simulink model "ThevinenIdentification_uding_ESCAndEst"  (R2021b)
settings: Solver=VariableStepAuto  StartTime=0.0  StopTime=300  FixedStep=0.01  MaxStep=1  RelTol=1e-4
undefined symbols (not defined in the file): sgn
libraries: simulink_extras x7, spsSeriesRLCBranchLib x4, spsBreakerLib x2, spsFourierLib x2, spsACVoltageSourceLib x1, simulink x1, spsGroundLib x1, spsControlledCurrentSourceLib x1, spsCurrentMeasurementLib x1, spsPowerLib x1, spsVoltageMeasurementLib x1, spspowerguiLib x1
settings Model: Creator=tahas  LastModifiedBy=tahas

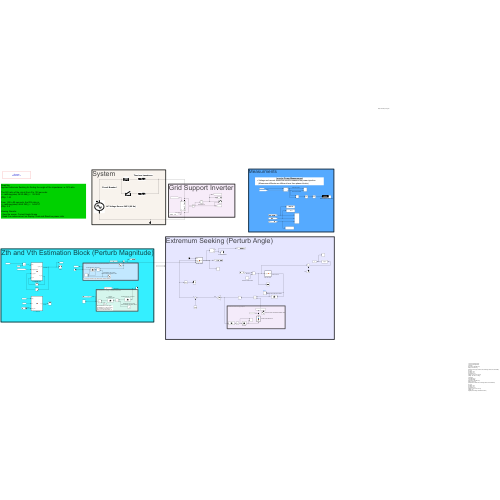
[thumbnail: Simulink's stored preview of the top-level diagram]
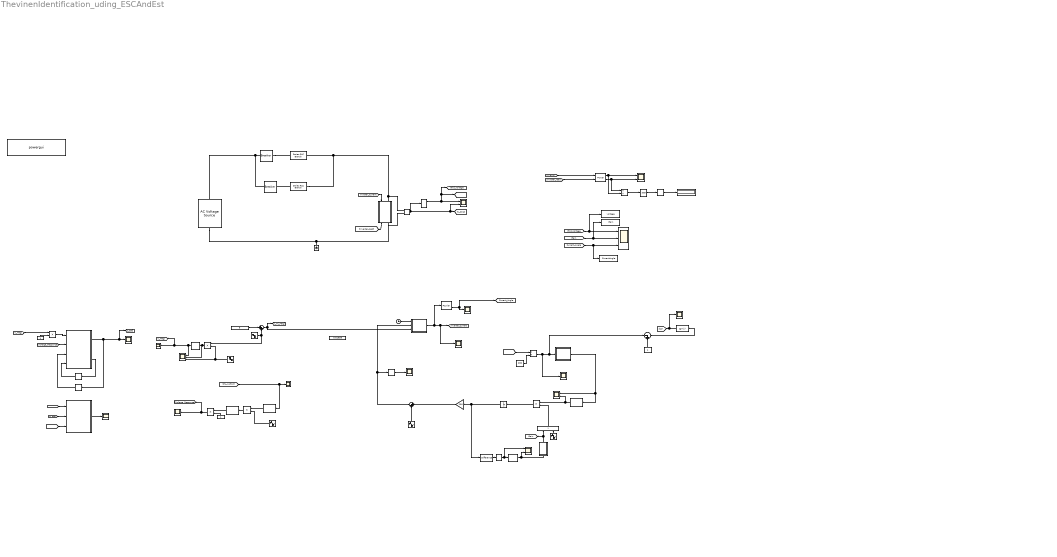
== system ThevinenIdentification_uding_ESCAndEst ==
  note: Zth and Vth Estimation Block (Perturb Magnitude)
  note: Grid Support Inverter (Current Source)
  note: After demodulation, the DC signal gets divided by 2, so we can multiply by 2 if needed (not needed here since input is also got divided by 2)
  note: Conditional Gain Change (Optional)
  note: System
  note: Measurments
  note: Extremum Seeking (Perturb Angle)
  note: Read Me:
      | Applies Extremum Seeking for finding the angle of the impedance i.e. R/X ratio.
      |
      | The R/X ratio of the circuit from 0 to 100 seconds:
      | >> rad2deg(atan(.343/0.484)) = 35.3243
      | |Zth|= 1.42
      |
      | From 105 to 90 seconds, the R/X ratio is:
      | >> rad2deg(atan(0.484/.343)) = 54.6757
      | |Zth|= 2.8
      |
      | Viewing Results:
      | - View the scope: Current Angle Scope
      | - Read the measurement on display: Real and Reactive power ratio
      |
      | Note:
      | Change filter to s/(s+1) and gain to 150 to visualize beautiful convergence
      | Change filter to s/(s+5) and gain to 200 to get quick convergence
  note: x=out.CurrentAngle.Time;
      | y=out.CurrentAngle.Data;
      | yyaxis left
      | h(1)=plot(x,y,'linewidth',2.0);
      | axis([13 34 -200 200])
      | ylabel('Current Angle','FontSize',32,'FontWeight','bold','Color','#0072BD')
      | ax = gca;
      | ax.XGrid = 'off';
      | ax.YGrid = 'on';
      | ax.FontSize = 32;
      | xticks([15 18 21 24 27 30 32])
      | yticks([ -180 -60 -30 0 180])
      | yyaxis right
      | x=out.Gain.Time;
      | y=out.Gain.Data;
      | h(2)=plot(x,y,'linewidth',2.0);
      | axis([13 34 -5 45])
      | ylabel('Gain','FontSize',32,'FontWeight','bold','Color','#D95319')
      | ax = gca;
      | ax.XGrid = 'off';
      | ax.YGrid = 'on';
      | ax.FontSize = 32;
      | xticks([15 18 21 24 27 30 33])
      | yticks([ 1 8])
      | legend('Current Angle','Demodulator Gain')
  note: Inverter Power Measurement
      | Voltage and current should be used to measure the power injection (Measuremnt Blocks are different here then phasor blocks)
  note: Circuit Breakerl
  note: Thevinen Impedance
  note: AC Voltage Source 245 V (60 Hz)
  note: For viewing the waveforms (the effect of filter and demodulation)
  note: Saving the 0.5 of ampliftude of applied perturbation
  note: The response on voltage of applied perturbation
  note: atan(.343/0.484) in degree
  " Intention: To separate DC part" : simulink_extras/Additional Linear/Transfer Fcn (with initial outputs)  N=[0 1]  D="[1  1]"  Y0=0  U0=0
  AC Voltage Source1 : spsACVoltageSourceLib/AC Voltage Source  Amplitude=245  Phase=0  Frequency=60  SampleTime=0  Measurements=None  BusType=swing  Pref=10e3  Qref=0  Qmin=-inf  Qmax=+inf
  Add1 : Sum  Inputs=|-+
  Atan1 : Trigonometry  Operator=atan
  Breaker1 : spsBreakerLib/Breaker  InitialState=1  SwitchingTimes=[105 195]  External=off  BreakerResistance=0.00000001  SnubberResistance=1e6  SnubberCapacitance=inf  Measurements=None  MoreParameters=on  NoBreakLoop=off
      settings: SourceProductBaseCode=PS
  Breaker3 : spsBreakerLib/Breaker  InitialState=0  SwitchingTimes=[100 200]  External=off  BreakerResistance=0.00000001  SnubberResistance=1e6  SnubberCapacitance=inf  Measurements=None  MoreParameters=on  NoBreakLoop=off
      settings: SourceProductBaseCode=PS
  Clock : Clock
  Complex to Magnitude-Angle : ComplexToMagnitudeAngle  Output=Magnitude
  "Conditional Gain Adjustment " : MATLAB Function  TreatAsAtomicUnit=on
  Current Angle Scope : Scope
  "Demodulation with the same signal as applied parturbation, Mag=1" : Sin  Frequency=10  SampleTime=0
  "Demodulation with the same signal as applied parturbation, Mag=1 " : Sin  Frequency=10  SampleTime=0
  Difference : simulink/Discrete/Difference  ICPrevInput=0  OutMin=[]  OutMax=[]  OutDataType=fixdt(1, 16)  OutScaling=2^-10  DoSatur=off
  Divide1 : Product  Inputs=*/
  Divide4 : Product  Inputs=*/
  Fcn2 : Fcn  Expr=sgn(u)
  Fourier at 60 Hz : spsFourierLib/Fourier  Freq=60  n=1  InInit=[0, 0]  Ts=0
      settings: SourceProductBaseCode=PS
  Fourier7 : spsFourierLib/Fourier  Freq=60  n=1  InInit=[0, 0]  Ts=0
      settings: SourceProductBaseCode=PS
  Gain : Gain  Gain=200
  Ground2 : spsGroundLib/Ground  LConnTagsString=a
  High pass filter (with initial outputs)1 : simulink_extras/Additional Linear/Transfer Fcn (with initial outputs)  N=[1 0]  D="[1  5]"  Y0=0  U0=0
  High pass filter with 1 rad cut off : simulink_extras/Additional Linear/Transfer Fcn (with initial outputs)  N=[1 0]  D="[1  1]"  Y0=0  U0=0
  Integrator1 : Integrator
  Inverter : Subsystem
  Low Pass : simulink_extras/Additional Linear/Transfer Fcn (with initial outputs)  N=[0 1]  D="[1  6]"  Y0=0  U0=0
  Low pass filter with 1 rad cut off : simulink_extras/Additional Linear/Transfer Fcn (with initial outputs)  N=[0 1]  D="[1  1]"  Y0=0  U0=0
  Normilizing voltage (peak) : Constant  Value=280
  P_Prev : Memory  InitialCondition=0.1
  Power : spsPowerLib/Power  Freq=60  Vinit=[1, 0]  Iinit=[1, 0]  Ts=0
      settings: SourceProductBaseCode=PS
  Product{1..3,5..7} (6 alike) : Product
  Radians to Degrees : simulink_extras/Transformations/Radians to Degrees
  Radians to Degrees2 : simulink_extras/Transformations/Radians to Degrees
  Real Power (watts)1 : Constant  Value=5
  Real Power (watts)2 : Constant
  Real Power (watts)3 : Constant
  Real Power (watts)4 : Constant  Value=0.61655
  "Real and Reactive power ratio " : Display
  Scope{1,5,12,14} (4 alike) : Scope  NumInputPorts=2
  Scope10 : Scope  NumInputPorts=3
  Scope{2..4,6..7,9,11} (7 alike) : Scope
  Scope15 : Scope  NumInputPorts=3
  Series RLC Branch1 : spsSeriesRLCBranchLib/Series RLC Branch  LConnTagsString=__new0  RConnTagsString=__new0  BranchType=RL  Resistance=12*0.343*40/100  Inductance=12*0.484/(2*pi*60) *40/100  SetiL0=off  InitialCurrent=0  Capacitance=1e-6  Setx0=off  InitialVoltage=0  Measurements=None
  Series RLC Branch7 : spsSeriesRLCBranchLib/Series RLC Branch  LConnTagsString=__new0  RConnTagsString=__new0  BranchType=RL  Resistance=6*0.484*40/100  Inductance=6*0.343/(2*pi*60)*40/100  SetiL0=off  InitialCurrent=0  Capacitance=1e-6  Setx0=off  InitialVoltage=0  Measurements=None
  Sine Wave (same as applied perturbation freq) : Sin  Frequency=5  SampleTime=0
  Sine Wave2 : Sin  Amplitude=0.01  Frequency=5  SampleTime=0
  Sine Wave5 : Sin  Amplitude=0.005  Frequency=10  SampleTime=0
  Sum1 : Sum  Inputs=|++
  Sum3 : Sum  Inputs=|++
  To Workspace : ToWorkspace  VariableName=voltage  SaveFormat=Timeseries  SampleTime=-1
  To Workspace1 : ToWorkspace  VariableName=Gain  SaveFormat=Timeseries  SampleTime=-1
  To Workspace2 : ToWorkspace  VariableName=CurrentAngle  SaveFormat=Timeseries  SampleTime=-1
  V1 : Scope
  V_th_Est Block : MATLAB Function  TreatAsAtomicUnit=on
  Volt_Var_Curve1 : MATLAB Function  TreatAsAtomicUnit=on
  Volt_Var_Curve3 : MATLAB Function  TreatAsAtomicUnit=on
  Voltage Measurement4 : spsVoltageMeasurementLib/Voltage Measurement  PhasorSimulation=off  OutputType=Complex  PSBequivalent=0
  Vref : Constant
  Z_Est : Scope
  Z_Prev1 : Memory  InitialCondition=0.1
  Zth Estimation Block : MATLAB Function  TreatAsAtomicUnit=on
  powergui : spspowerguiLib/powergui  SimulationMode=Discrete  SampleTime=1/60/100  frequency=60  Iterations=50  frequencyindice=60  Pbase=100e6  ErrMax=1e-4  UnitsV=kV  UnitsW=MW  buscounter=0  FunctionMessages=off  echomessages=off  EnableUseOfTLC=off  CurrentSourceSwitches=off  DisableSnubberDevices=off  DisableRonSwitches=off  DisableVfSwitches=off  DisplayEquations=off  AutomaticDiscreteSolvers=off  SolverType=Tustin  Interpol=off  ExternalGateDelay=off  methode=off  Ts=0  x0status=blocks  SPID=off  SwTol=0  HookPort=off  NonlinearTolerance=1e-4  nMaxIteration=100  ContinueOnMaxIteration=off  RestoreLinks=warning  ResistiveCurrentMeasurement=off  Frange=[0:2:500]  Ylog=off  Xlog=on  ShowGrid=off  save=off  variable=ZData  structure=0  ZoomFFT=on  StartTime=0.0  cycles=1  DisplayStyle=1  fundamental=60  FreqAxis=off  MaxFrequency=1000  frequencyindicesteady=1  RmsSteady=1  display=off
  tag scope: Current_Angle=global, Gain=global, Grid_Voltage=global, Inverter_Current=global, sign=global
  wires:
  Fcn2/1 -> Scope9/1, [sign]
  Volt_Var_Curve3/1(cost) -> High pass filter (with initial outputs)1/1, Scope5/1  "Reactive Power inj"
  Product1/1 -> Integrator1/1
  Vref/1 -> Add1/2
  [PU_V_Grid] -> Divide1/1  "Maximizing"
  Sine Wave2/1 -> Sum1/2
  Add1/1 -> Fcn2/1
  Clock/1 -> Volt_Var_Curve1/1(time)
  Volt_Var_Curve1/1(current) -> Fourier7/1, Scope3/1, [Inverter_Current]  "Reactive Power inj"
  Voltage Measurement4/1 -> Fourier at 60 Hz/1, Scope1/2, [V_Grid]
  Inverter/1(Out1) -> [Inverter_read]  "Current Reading"
  [Inverter_Current] -> Inverter/1(In1)  "Current Seeting"
  Sum1/1 -> Volt_Var_Curve1/2(angle), Radians to Degrees/1  "pf"
  [V_Grid] -> Power/1  "voltage"
  [Inverter_read] -> Power/2
  High pass filter (with initial outputs)1/1 -> Scope5/2, Product1/1
  Fourier7/2 -> [Current_Angle], Current Angle Scope/1
  Integrator1/1 -> Gain/1, Difference/1
  Gain/1 -> Sum1/1  "Gain"
  Low Pass/1 -> "Conditional Gain Adjustment "/1(differ), Scope12/2
  Complex to Magnitude-Angle/1 -> Low Pass/1, Scope12/1
  Difference/1 -> Complex to Magnitude-Angle/1
  Radians to Degrees/1 -> Scope4/1
  Fourier at 60 Hz/1 -> [Grid_Voltage], [PU_V_Grid], Scope1/1
  [Gain] -> To Workspace1/1, Scope15/2
  [Grid_Voltage] -> To Workspace/1, Scope15/1
  [Current_Angle] -> To Workspace2/1, Scope15/3
  "Conditional Gain Adjustment "/1(Gain) -> Product7/1, [Gain]
  Sine Wave (same as applied perturbation freq)/1 -> Product7/2
  Product7/1 -> Product1/2
  Power/1 -> Divide4/2, Scope14/1  "Real Power Injected"
  Atan1/1 -> Radians to Degrees2/1
  Radians to Degrees2/1 -> "Real and Reactive power ratio "/1
  Power/2 -> Divide4/1, Scope14/2  "Reactive Power Injected"
  Divide4/1 -> Atan1/1
  Normilizing voltage (peak)/1 -> Divide1/2
  Divide1/1 -> Scope6/1, Add1/1, Volt_Var_Curve3/1(U_grid)
  Sum3/1 -> Volt_Var_Curve1/3(I_mag), [I_Inj_Mag]
  Real Power (watts)1/1 -> Sum3/1
  Sine Wave5/1 -> Sum3/2, Product5/1
  Product5/1 -> Scope10/2, Low pass filter with 1 rad cut off/1
  Low pass filter with 1 rad cut off/1 -> Scope11/1, [I_Mag], Scope10/1
  Zth Estimation Block/1(th_hat_next) -> Z_Prev1/1, [Z_Est], Z_Est/1  "Z_estimatej"
  Product3/1 -> " Intention: To separate DC part"/1
  Real Power (watts)2/1 -> Product6/2
  High pass filter with 1 rad cut off/1 -> Product3/1
  " Intention: To separate DC part"/1 -> Product6/1
  [PU_V_Grid] -> High pass filter with 1 rad cut off/1, V1/1  "Grid Voltage"
  Product6/1 -> Scope7/1, [Voltage_Response]
  Z_Prev1/1 -> Zth Estimation Block/3(th_hat_prev)
  [Voltage_Response] -> Zth Estimation Block/2(VoltageResponse)
  P_Prev/1 -> Zth Estimation Block/4(P_prev)
  Zth Estimation Block/2(P_next) -> P_Prev/1
  "Demodulation with the same signal as applied parturbation, Mag=1 "/1 -> Product3/2
  [I_Mag] -> Product2/1
  Real Power (watts)3/1 -> Product2/2
  Product2/1 -> Zth Estimation Block/1(IMag)
  "Demodulation with the same signal as applied parturbation, Mag=1"/1 -> Scope10/3, Product5/2
  [PU_V_Grid] -> V_th_Est Block/3(Meas_Volt)  "Grid Voltage"
  V_th_Est Block/1(V_th) -> Scope2/1  "estimatej"
  [Z_Est] -> V_th_Est Block/2(Zth)
  [I_Inj_Mag] -> V_th_Est Block/1(IMag)
  connections:
  Ground2/LConn1 -- Voltage Measurement4/LConn2 -- Inverter/RConn1 -- AC Voltage Source1/LConn1
  Breaker3/LConn1 -- AC Voltage Source1/RConn1 -- Breaker1/LConn1
  Series RLC Branch1/LConn1 -- Breaker3/RConn1
  Breaker1/RConn1 -- Series RLC Branch7/LConn1
  Series RLC Branch1/RConn1 -- Inverter/LConn1 -- Voltage Measurement4/LConn1 -- Series RLC Branch7/RConn1

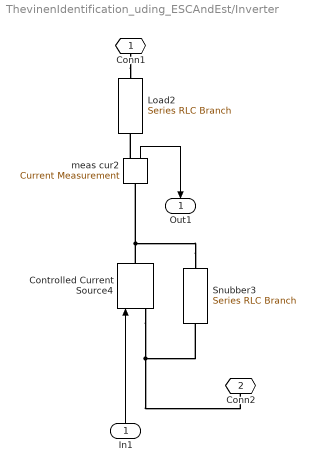
== system ThevinenIdentification_uding_ESCAndEst/Inverter ==
  In1 : Inport
  Controlled Current Source4 : spsControlledCurrentSourceLib/Controlled Current Source  Initialize=on  Source_Type=AC  Amplitude=16.6  Phase=-30  Frequency=60  Measurements=None
  Load2 : spsSeriesRLCBranchLib/Series RLC Branch  LConnTagsString=__new0  RConnTagsString=__new0  BranchType=R  Resistance=16  Inductance=1e-3  SetiL0=off  InitialCurrent=0  Capacitance=1e-6  Setx0=off  InitialVoltage=0  Measurements=None
  Snubber3 : spsSeriesRLCBranchLib/Series RLC Branch  LConnTagsString=__new0  RConnTagsString=__new0  BranchType=R  Resistance=1e6  Inductance=1e-3  SetiL0=off  InitialCurrent=0  Capacitance=1e-6  Setx0=off  InitialVoltage=0  Measurements=None
  meas cur2 : spsCurrentMeasurementLib/Current Measurement  PhasorSimulation=off  OutputType=Complex  PSBequivalent=0
  Conn1 : PMIOPort  Side=Left
  Conn2 : PMIOPort  Port=2  Side=Right
  Out1 : Outport
  wires:
  In1/1 -> Controlled Current Source4/1
  meas cur2/1 -> Out1/1
  connections:
  Conn1/RConn1 -- Load2/LConn1
  meas cur2/RConn1 -- Load2/RConn1
  Snubber3/LConn1 -- meas cur2/LConn1 -- Controlled Current Source4/RConn1
  Snubber3/RConn1 -- Conn2/RConn1 -- Controlled Current Source4/LConn1

== matlab function ThevinenIdentification_uding_ESCAndEst/Volt_Var_Curve1 ==
  data: time input; current output; angle input; I_mag input
function current = fcn(time,angle,I_mag)

current= I_mag*sin(2*pi*60*time - angle);

== matlab function ThevinenIdentification_uding_ESCAndEst/Zth Estimation Block ==
  data: IMag input; th_hat_next output; VoltageResponse input; th_hat_prev input; P_next output; P_prev input

function [th_hat_next, P_next] = SimulinkEstimateOnline(IMag, VoltageResponse,th_hat_prev, P_prev)
    % Apply low pass filter
    Isinthe = IMag.^1; % Assuming IMag is scalar

    % Correct for high pass filter degain
    z = VoltageResponse * 1.005; % Assuming VoltageResponse is scalar % correcting filter attenuation

    % Check if initial state is provided, otherwise initialize
    if isempty(th_hat_prev)
        th_hat_prev = 0.1; % Adjust initial value as needed
        P_prev = eye(1); % Initial P matrix
    end

    % Define parameters
    sigma = 0.0001; % Standard deviation for noise

    % Recursive Weighted Least Squares (RWLS) algorithm
    h_k_plus1 = [Isinthe];
    Kw_kplus1 = (P_prev * h_k_plus1') / (h_k_plus1 * P_prev * h_k_plus1' + sigma^2);
    th_hat_next = th_hat_prev + Kw_kplus1 * (z - h_k_plus1 * th_hat_prev);
    P_next = (1/0.99)*(P_prev - Kw_kplus1 * h_k_plus1 * P_prev); % With forgetting factor

end

== matlab function ThevinenIdentification_uding_ESCAndEst/Conditional Gain Adjustment  ==
  data: differ input; Gain output
function Gain = fcn(differ)

if (differ < 10e-8)
    Gain=8;
else
    Gain=1;
end

== matlab function ThevinenIdentification_uding_ESCAndEst/Volt_Var_Curve3 ==
  data: U_grid input; cost output
function cost = fcn(U_grid)

cost= (U_grid);

== matlab function ThevinenIdentification_uding_ESCAndEst/V_th_Est Block ==
  data: IMag input; V_th output; Zth input; Meas_Volt input

function V_th = SimulinkEstimateOnline(IMag, Zth, Meas_Volt)
    V_th = abs(Meas_Volt)- abs(IMag)* abs(Zth);
end
